simulink model "fft_analysis"  (R2020b)
settings: Solver=FixedStepDiscrete  StartTime=0.0  StopTime=0.01  RelTol=1e-3
undefined symbols (not defined in the file or in its folder): mp
libraries: hdlsllib x7, simulink x4, dsphdlxfrm x1, dspsigops x1
settings Model: DataTypeOverride=Off  Creator=Ross  LastModifiedBy=conno
settings DataIOCC: SaveOutput=off  SaveTime=off  ReturnWorkspaceOutputs=off
settings OptimizationCC: BlockReduction=off  ConditionallyExecuteInputs=off  DefaultParameterBehavior=Inlined
settings DebuggingCC: ReadBeforeWriteMsg=DisableAll  WriteAfterWriteMsg=DisableAll  WriteAfterReadMsg=DisableAll  AlgebraicLoopMsg=error  MultiTaskDSMMsg=none  SingleTaskRateTransMsg=error  PregeneratedLibrarySubsystemCodeDiagnostic=none  ArithmeticOperatorsInVariantConditions=warning
settings HardwareCC: ProdBitPerPointer=32  ProdBitPerSizeT=32  ProdBitPerPtrDiffT=32  ProdLargestAtomicFloat=None  ProdIntDivRoundTo=Undefined  ProdEndianess=Unspecified  ProdWordSize=32  ProdHWDeviceType=ASIC/FPGA->ASIC/FPGA  TargetBitPerPointer=64  TargetBitPerSizeT=64  TargetBitPerPtrDiffT=64  TargetLongLongMode=on  TargetIntDivRoundTo=Zero  TargetEndianess=LittleEndian  TargetWordSize=64  TargetHWDeviceType=Custom Processor->MATLAB Host Computer  ProdEqTarget=off
settings ModelReferenceCC: UpdateModelReferenceTargets=IfOutOfDate
settings SFSimCC: SFSimEcho=off  SimUseLocalCustomCode=off  CustomCodeUndefinedFunction=UseInterfaceOnly
settings RTWCC: RTWUseLocalCustomCode=off

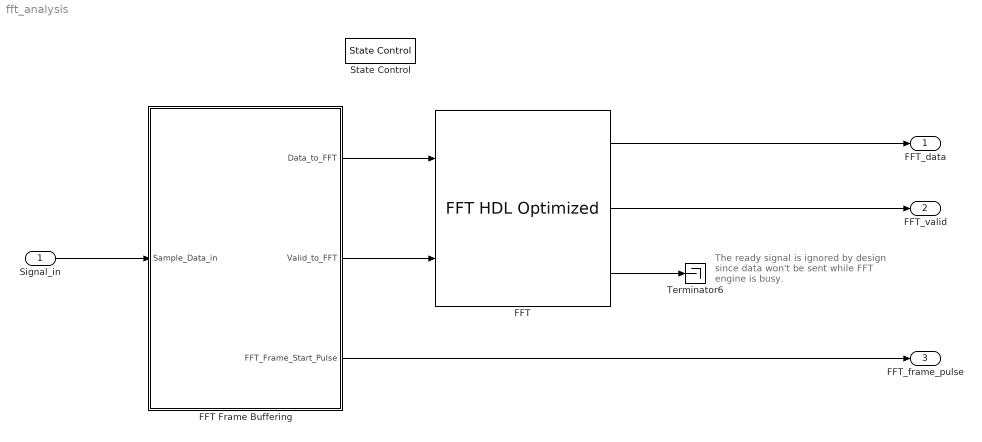
== system fft_analysis ==
  note: The ready signal is ignored by design
      | since data won't be sent while FFT
      | engine is busy.
  Signal_in : Inport  OutDataTypeStr=fixdt(1,24,23)  PortDimensions=1  SampleTime=[2.0833333333333333e-05,0]
  FFT : dsphdlxfrm/FFT HDL Optimized  FFTLength=mp.FFT_size  Architecture=Burst Radix 2  ComplexMultiplication=Use 4 multipliers and 2 adders  BitReversedOutput=off  BitReversedInput=off  Normalize=off  SimulateUsing=Code generation  RoundingMethod=Floor  ResetInputPort=off  StartOutputPort=off  EndOutputPort=off
      settings: SourceProductBaseCode=DS
  FFT Frame Buffering : Subsystem
  State Control : StateControl  StateControl=Synchronous
  Terminator6 : Terminator
  FFT_data : Outport  PortDimensions=1  SampleTime=[1.6276041666666666e-07,0]  VectorParamsAs1DForOutWhenUnconnected=off
      settings: SignalType=complex
  FFT_valid : Outport  Port=2  OutDataTypeStr=boolean  PortDimensions=1  SampleTime=[1.6276041666666666e-07,0]  VectorParamsAs1DForOutWhenUnconnected=off
  FFT_frame_pulse : Outport  Port=3  OutDataTypeStr=boolean  PortDimensions=1  SampleTime=[1.6276041666666666e-07,0]  VectorParamsAs1DForOutWhenUnconnected=off
  wires:
  FFT/3 -> Terminator6/1
  FFT Frame Buffering/3(FFT_Frame_Start_Pulse) -> FFT_frame_pulse/1
  Signal_in/1 -> FFT Frame Buffering/1(Sample_Data_in)
  FFT Frame Buffering/2(Valid_to_FFT) -> FFT/2
  FFT Frame Buffering/1(Data_to_FFT) -> FFT/1
  FFT/2 -> FFT_valid/1
  FFT/1 -> FFT_data/1

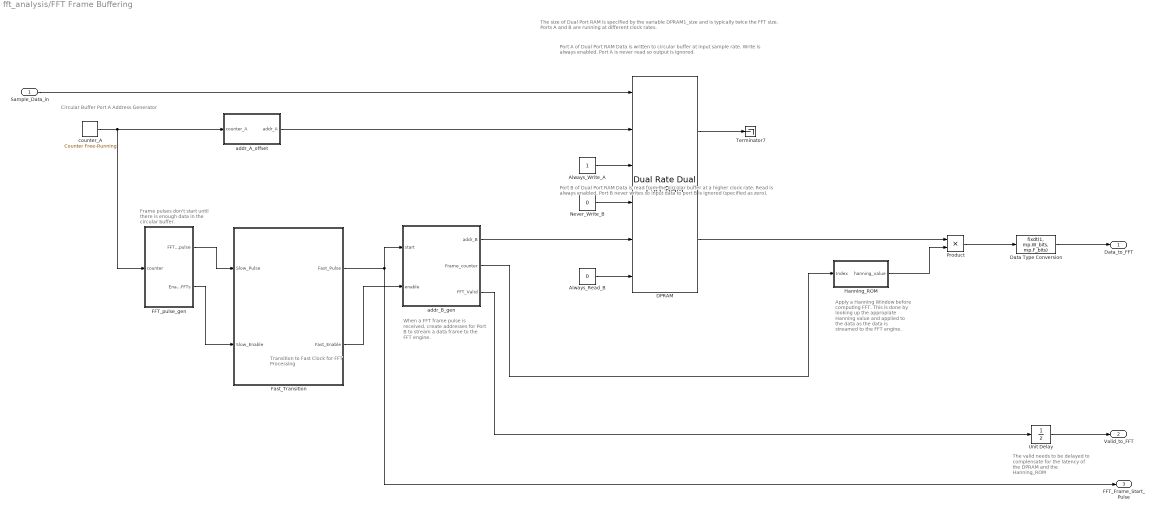
== system fft_analysis/FFT Frame Buffering ==
  note: Port B of Dual Port RAM
      |
      | Data is read from the circular buffer at a higher clock rate.
      | Read is always enabled.  Port B never writes so input data to port B
      | is ignored (specified as zero).
  note: Transition to
      | Fast Clock
      | for FFT Processing
  note: Port A of Dual Port RAM
      |
      | Data is written to circular buffer at input sample rate.
      | Write is always enabled.  Port A is never read so output is ignored.
  note: Circular Buffer
      | Port A Address Generator
  note: The size of Dual Port RAM is specified by the variable DPRAM1_size
      | and is typically twice the FFT size.  Ports A and B are running at different clock rates.
  note: Frame pulses don't start
      | until there is enough data
      | in the circular buffer.
  note: Apply a Hanning Window
      | before computing FFT.  This
      | is done by looking up the
      | appropiate Hanning value
      | and applied to the data as the
      | data is streamed to the
      | FFT engine.
  note: When a FFT frame pulse
      | is received, create addresses for
      | Port B to stream a data frame
      | to the FFT engine.
  note: The valid needs to be delayed
      | to complensate for the latency
      | of the DPRAM and the
      | Hanning_ROM
  Sample_Data_in : Inport
  Always_Read_B : Constant  Value=0  OutDataTypeStr=boolean  SampleTime=mp.Ts/mp.SysRate_Upsample_Factor
  Always_Write_A : Constant  OutDataTypeStr=boolean  SampleTime=mp.Ts
  DPRAM : hdlsllib/HDL RAMs/Dual Rate Dual Port RAM  ram_size=mp.DPRAM1_address_size
      settings: SourceProductBaseCode=SL
  Data Type Conversion : DataTypeConversion  OutDataTypeStr=fixdt(1, mp.W_bits, mp.F_bits)
  FFT_pulse_gen : Subsystem
  Fast_Transition : Subsystem
  Hanning_ROM : Subsystem
  Never_Write_B : Constant  Value=0  OutDataTypeStr=fixdt(1,24,23)  SampleTime=mp.Ts/mp.SysRate_Upsample_Factor
  Product : Product
  Terminator7 : Terminator
  Unit Delay : UnitDelay  SampleTime=-1  HasFrameUpgradeWarning=on
  addr_A_offset : Subsystem
  addr_B_gen : Subsystem
  counter_A : simulink/Sources/Counter Free-Running  NumBits=mp.DPRAM1_address_size  tsamp=mp.Ts
  Data_to_FFT : Outport  VectorParamsAs1DForOutWhenUnconnected=off
  Valid_to_FFT : Outport  Port=2  VectorParamsAs1DForOutWhenUnconnected=off
  FFT_Frame_Start_Pulse : Outport  Port=3  VectorParamsAs1DForOutWhenUnconnected=off
  wires:
  Unit Delay/1 -> Valid_to_FFT/1
  Fast_Transition/2(Fast_Enable) -> addr_B_gen/2(enable)
  FFT_pulse_gen/2(Enable_FFTs) -> Fast_Transition/2(Slow_Enable)
  FFT_pulse_gen/1(FFT_start_pulse) -> Fast_Transition/1(Slow_Pulse)
  Fast_Transition/1(Fast_Pulse) -> FFT_Frame_Start_Pulse/1, addr_B_gen/1(start)
  Data Type Conversion/1 -> Data_to_FFT/1
  Hanning_ROM/1(hanning_value) -> Product/2
  DPRAM/2 -> Product/1
  Product/1 -> Data Type Conversion/1
  addr_B_gen/2(Frame_counter) -> Hanning_ROM/1(Index)
  addr_A_offset/1(addr_A) -> DPRAM/2
  Sample_Data_in/1 -> DPRAM/1
  counter_A/1 -> FFT_pulse_gen/1(counter), addr_A_offset/1(counter_A)
  addr_B_gen/1(addr_B) -> DPRAM/5
  addr_B_gen/3(FFT_Valid) -> Unit Delay/1
  DPRAM/1 -> Terminator7/1
  Always_Read_B/1 -> DPRAM/6
  Never_Write_B/1 -> DPRAM/4
  Always_Write_A/1 -> DPRAM/3

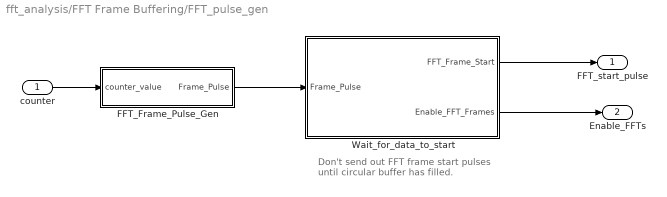
== system fft_analysis/FFT Frame Buffering/FFT_pulse_gen ==
  note: Don't send out FFT frame start pulses
      | until circular buffer has filled.
  counter : Inport
  FFT_Frame_Pulse_Gen : Subsystem
  Wait_for_data_to_start : Subsystem
  FFT_start_pulse : Outport  VectorParamsAs1DForOutWhenUnconnected=off
  Enable_FFTs : Outport  Port=2  VectorParamsAs1DForOutWhenUnconnected=off
  wires:
  FFT_Frame_Pulse_Gen/1(Frame_Pulse) -> Wait_for_data_to_start/1(Frame_Pulse)
  Wait_for_data_to_start/2(Enable_FFT_Frames) -> Enable_FFTs/1
  Wait_for_data_to_start/1(FFT_Frame_Start) -> FFT_start_pulse/1
  counter/1 -> FFT_Frame_Pulse_Gen/1("counter_value ")

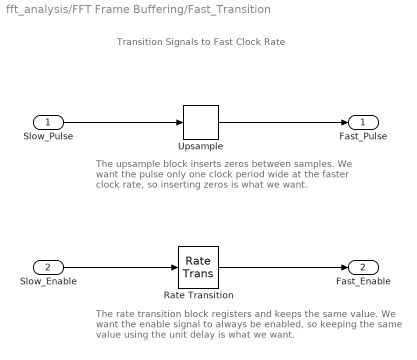
== system fft_analysis/FFT Frame Buffering/Fast_Transition ==
  note: The rate transition block registers and keeps the same
      | value.  We want the enable signal to always be enabled,
      | so keeping the same value using the unit delay is what we want.
  note: Transition Signals to Fast Clock Rate
  note: The upsample block inserts zeros between samples.
      | We want the pulse only one clock period wide at the
      | faster clock rate, so inserting zeros is what we want.
  Slow_Pulse : Inport
  Slow_Enable : Inport  Port=2
  Rate Transition : RateTransition  OutPortSampleTimeOpt=Multiple of input port sample time  OutPortSampleTimeMultiple=1/mp.SysRate_Upsample_Factor
  Upsample : dspsigops/Upsample  N=mp.SysRate_Upsample_Factor  phase=0  RateOptions=Allow multirate processing  ic=0  mode=Unused parameter value
  Fast_Pulse : Outport
  Fast_Enable : Outport  Port=2
  wires:
  Upsample/1 -> Fast_Pulse/1
  Slow_Enable/1 -> Rate Transition/1
  Rate Transition/1 -> Fast_Enable/1
  Slow_Pulse/1 -> Upsample/1

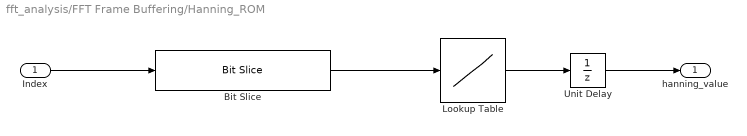
== system fft_analysis/FFT Frame Buffering/Hanning_ROM ==
  Index : Inport
  Bit Slice : hdlsllib/Logic and Bit Operations/Bit Slice  lidx=log2(mp.FFT_size) - 1  ridx=0
      settings: SourceProductBaseCode=SL
  Lookup Table : Lookup_n-D  NumberOfTableDimensions=1  BreakpointsForDimension1=[0:mp.FFT_size-1]  IndexSearchMethod=Evenly spaced points  Table=hanning(mp.FFT_size)  InterpMethod=Flat  ExtrapMethod=Clip  DiagnosticForOutOfRangeInput=Warning  UseLastTableValue=on  OutDataTypeStr=fixdt(1,24,23)  RndMeth=Simplest  InputSameDT=on
  Unit Delay : UnitDelay  SampleTime=-1  HasFrameUpgradeWarning=on
  hanning_value : Outport  VectorParamsAs1DForOutWhenUnconnected=off
  wires:
  Bit Slice/1 -> Lookup Table/1
  Lookup Table/1 -> Unit Delay/1
  Index/1 -> Bit Slice/1
  Unit Delay/1 -> hanning_value/1

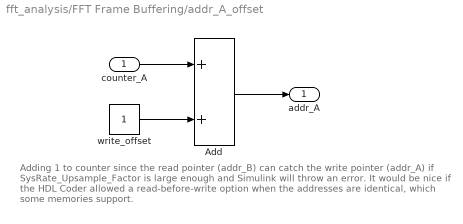
== system fft_analysis/FFT Frame Buffering/addr_A_offset ==
  note: Adding 1 to counter since the read pointer (addr_B) can catch the write pointer (addr_A)
      | if SysRate_Upsample_Factor is large enough and Simulink will throw an error.
      | It would be nice if the HDL Coder allowed a read-before-write option when
      | the addresses are identical, which some memories support.
  counter_A : Inport
  Add : Sum  OutDataTypeStr=fixdt(0,mp.DPRAM1_address_size,0)
  write_offset : Constant  OutDataTypeStr=fixdt(0,mp.DPRAM1_address_size,0)  SampleTime=mp.Ts
  addr_A : Outport  VectorParamsAs1DForOutWhenUnconnected=off
  wires:
  counter_A/1 -> Add/1
  Add/1 -> addr_A/1
  write_offset/1 -> Add/2

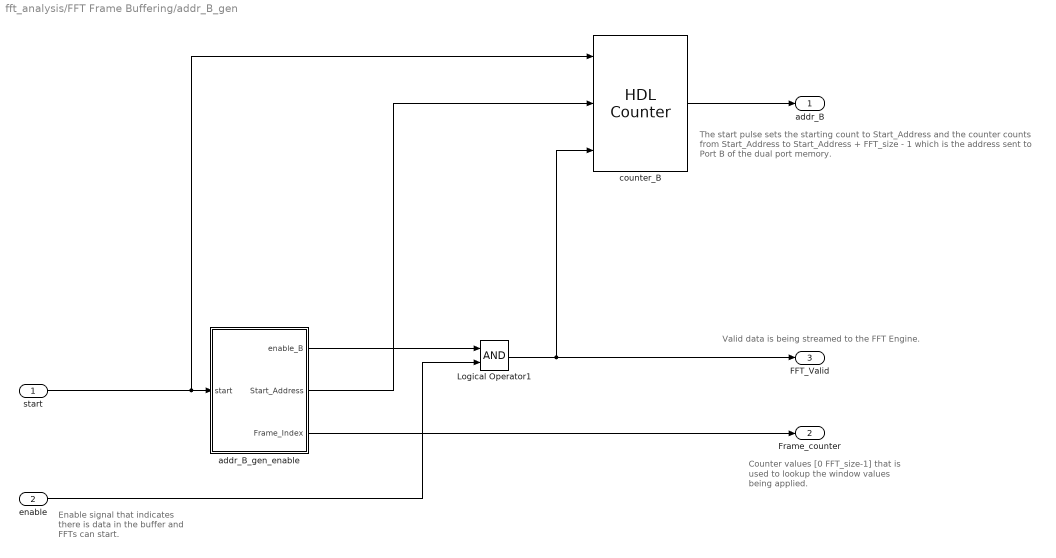
== system fft_analysis/FFT Frame Buffering/addr_B_gen ==
  note: The start pulse sets the starting count to Start_Address
      |  and the counter counts from Start_Address to Start_Address + FFT_size - 1
      | which is the address sent to Port B of the dual port memory.
  note: Enable signal that indicates
      | there is data in the buffer
      | and FFTs can start.
  note: Valid data is being streamed to the FFT Engine.
  note: Counter values [0 FFT_size-1] that
      | is used to lookup the window values
      | being applied.
  start : Inport
  enable : Inport  Port=2
  Logical Operator1 : Logic  AllPortsSameDT=off  OutDataTypeStr=boolean
  addr_B_gen_enable : Subsystem
  counter_B : hdlsllib/Sources/HDL Counter  CountType=Free running  CountInit=mp.DPRAM1_size-10  CountStep=1  CountMax=1024  CountFromType=Initial value  CountFrom=mp.DPRAM1_size-10  CountResetPort=off  CountLoadPort=on  CountEnbPort=on  CountDirPort=off  CountDataType=Unsigned  CountWordLen=mp.DPRAM1_address_size  CountFracLen=0  CountSampTime=1
  addr_B : Outport  VectorParamsAs1DForOutWhenUnconnected=off
  Frame_counter : Outport  Port=2  VectorParamsAs1DForOutWhenUnconnected=off
  FFT_Valid : Outport  Port=3  VectorParamsAs1DForOutWhenUnconnected=off
  wires:
  Logical Operator1/1 -> FFT_Valid/1, counter_B/3
  addr_B_gen_enable/3(Frame_Index) -> Frame_counter/1
  enable/1 -> Logical Operator1/2
  addr_B_gen_enable/2(Start_Address) -> counter_B/2
  addr_B_gen_enable/1(enable_B) -> Logical Operator1/1
  start/1 -> addr_B_gen_enable/1(start), counter_B/1
  counter_B/1 -> addr_B/1

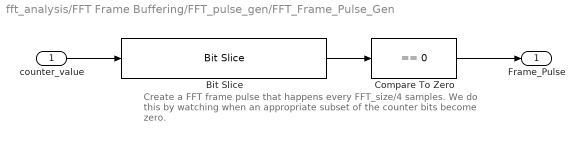
== system fft_analysis/FFT Frame Buffering/FFT_pulse_gen/FFT_Frame_Pulse_Gen ==
  note: Create a FFT frame pulse that happens every FFT_size/4 samples.
      | We do this by watching when an appropriate subset of the counter bits
      | become zero.
  "counter_value " : Inport
  Bit Slice : hdlsllib/Logic and Bit Operations/Bit Slice  lidx=log2(mp.FFT_frame_shift)-1  ridx=0
      settings: SourceProductBaseCode=SL
  Compare To Zero : simulink/Logic and Bit Operations/Compare To Zero  relop===  OutDataTypeStr=boolean
  Frame_Pulse : Outport  VectorParamsAs1DForOutWhenUnconnected=off
  wires:
  Bit Slice/1 -> Compare To Zero/1
  Compare To Zero/1 -> Frame_Pulse/1
  "counter_value "/1 -> Bit Slice/1

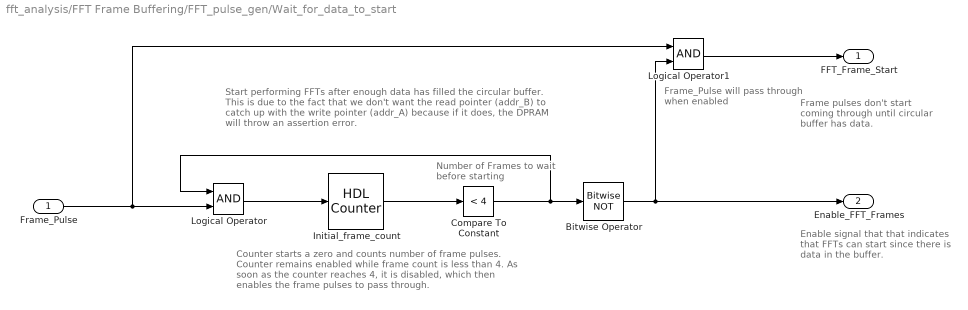
== system fft_analysis/FFT Frame Buffering/FFT_pulse_gen/Wait_for_data_to_start ==
  note: Enable signal that that indicates
      | that FFTs can start since there is
      | data in the buffer.
  note: Start performing FFTs after enough data has filled the circular buffer.
      | This is due to the fact that we don't want the read pointer (addr_B)
      | to catch up with the write pointer (addr_A) because if it does,
      | the DPRAM will throw an assertion error.
  note: Number of Frames
      | to wait before starting
  note: Frame_Pulse
      | will pass through
      | when enabled
  note: Counter starts a zero and counts number of frame pulses.
      | Counter remains enabled while frame count is less than 4.
      | As soon as the counter reaches 4, it is disabled, which then
      | enables the frame pulses to pass through.
  note: Frame pulses don't start
      | coming through until
      | circular buffer has data.
  Frame_Pulse : Inport
  Bitwise Operator : simulink/Logic and Bit Operations/Bitwise Operator  logicop=NOT  UseBitMask=off  BitMask=bin2dec('11011001')  BitMaskRealWorld=Stored Integer
  Compare To Constant : simulink/Logic and Bit Operations/Compare To Constant  relop=<  const=4  OutDataTypeStr=boolean
  Initial_frame_count : hdlsllib/Sources/HDL Counter  CountType=Count limited  CountInit=0  CountStep=1  CountMax=4  CountFromType=Specify  CountFrom=0  CountResetPort=off  CountLoadPort=off  CountEnbPort=on  CountDirPort=off  CountDataType=Unsigned  CountWordLen=5  CountFracLen=0  CountSampTime=1
  Logical Operator : Logic  AllPortsSameDT=off  OutDataTypeStr=boolean
  Logical Operator1 : Logic  AllPortsSameDT=off  OutDataTypeStr=boolean
  FFT_Frame_Start : Outport  VectorParamsAs1DForOutWhenUnconnected=off
  Enable_FFT_Frames : Outport  Port=2  VectorParamsAs1DForOutWhenUnconnected=off
  wires:
  Bitwise Operator/1 -> Logical Operator1/2, Enable_FFT_Frames/1
  Compare To Constant/1 -> Logical Operator/1, Bitwise Operator/1
  Logical Operator/1 -> Initial_frame_count/1
  Initial_frame_count/1 -> Compare To Constant/1
  Frame_Pulse/1 -> Logical Operator1/1, Logical Operator/2
  Logical Operator1/1 -> FFT_Frame_Start/1

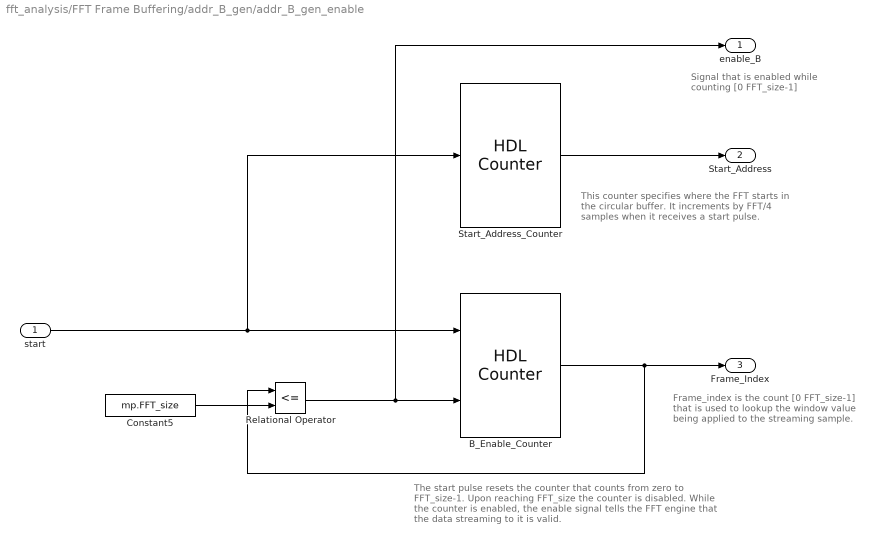
== system fft_analysis/FFT Frame Buffering/addr_B_gen/addr_B_gen_enable ==
  note: The start pulse resets the counter that counts
      | from zero to FFT_size-1.  Upon reaching FFT_size
      | the counter is disabled.  While the counter is enabled,
      | the enable signal tells the FFT engine that the data streaming
      | to it is valid.
  note: This counter specifies where the FFT starts
      | in the circular buffer.  It increments by FFT/4
      | samples when it receives a start pulse.
  note: Frame_index is the count [0 FFT_size-1]
      | that is used to lookup the window value
      | being applied to the streaming sample.
  note: Signal that is enabled while
      | counting [0 FFT_size-1]
  start : Inport
  B_Enable_Counter : hdlsllib/Sources/HDL Counter  CountType=Count limited  CountInit=0  CountStep=1  CountMax=mp.FFT_size  CountFromType=Specify  CountFrom=0  CountResetPort=on  CountLoadPort=off  CountEnbPort=on  CountDirPort=off  CountDataType=Unsigned  CountWordLen=mp.DPRAM1_address_size  CountFracLen=0  CountSampTime=1
  Constant5 : Constant  Value=mp.FFT_size  OutDataTypeStr=fixdt(0,mp.FFT_size_Nbits,0)  SampleTime=mp.Ts/mp.SysRate_Upsample_Factor
  Relational Operator : RelationalOperator  Operator=<=  OutDataTypeStr=boolean  ZeroCross=off  RndMeth=Nearest
  Start_Address_Counter : hdlsllib/Sources/HDL Counter  CountType=Free running  CountInit=0  CountStep=mp.FFT_frame_shift  CountMax=25  CountFromType=Initial value  CountFrom=0  CountResetPort=off  CountLoadPort=off  CountEnbPort=on  CountDirPort=off  CountDataType=Unsigned  CountWordLen=mp.DPRAM1_address_size  CountFracLen=0  CountSampTime=1
  enable_B : Outport  VectorParamsAs1DForOutWhenUnconnected=off
  Start_Address : Outport  Port=2  VectorParamsAs1DForOutWhenUnconnected=off
  Frame_Index : Outport  Port=3  VectorParamsAs1DForOutWhenUnconnected=off
  wires:
  Start_Address_Counter/1 -> Start_Address/1
  start/1 -> Start_Address_Counter/1, B_Enable_Counter/1
  B_Enable_Counter/1 -> Relational Operator/1, Frame_Index/1
  Constant5/1 -> Relational Operator/2
  Relational Operator/1 -> B_Enable_Counter/2, enable_B/1
